simulink model "RPEM_16_12_2005prueba"  (Simulink 5.0)
settings: Solver=ode45  StartTime=0.0  StopTime=10.0  RelTol=1e-3
undefined symbols (not defined in the file): ts
libraries: simulink x5
settings Model: LastModifiedBy=LeO

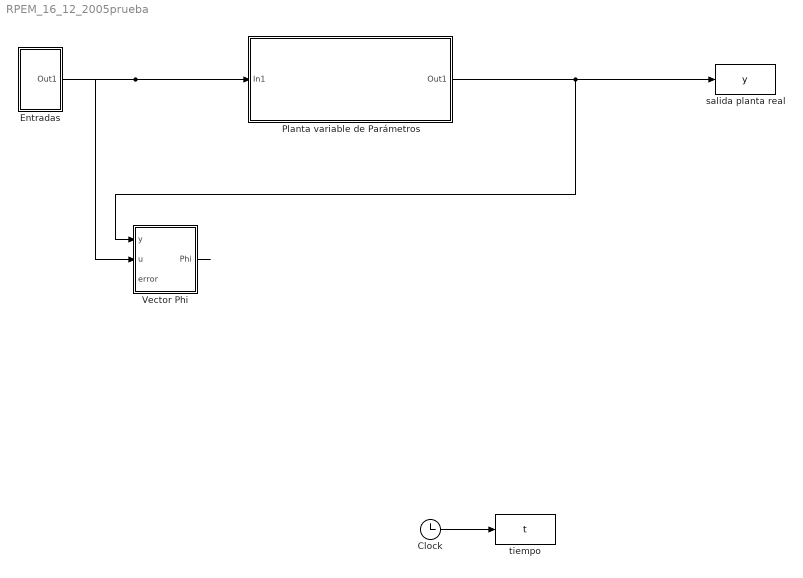
== system RPEM_16_12_2005prueba ==
  Clock : Clock
      settings: Decimation=10
  Entradas : Subsystem
  Planta variable de Parámetros : Subsystem  mask{ruido=0.05, tiempo1=40}
      mask prompts: tiempo1 "tiempo de movimiento de parametros de la planta"
  Vector Phi : Subsystem  mask{nu=1, ny=3, ne=1, nk=1}
      mask prompts: nu "Nº de u tomadas"; ny "Nº de y tomadas"; ne "Nº de errores tomados"; nk "Nº de retardo"
  salida planta real : ToWorkspace  VariableName=y  SampleTime=ts  SaveFormat=Array
  "tiempo " : ToWorkspace  VariableName=t  SampleTime=ts  SaveFormat=Array
  wires:
  Entradas/1(Out1) -> Planta variable de Parámetros/1(In1), Vector Phi/2(u)
  Clock/1 -> "tiempo "/1
  Planta variable de Parámetros/1(Out1) -> salida planta real/1, Vector Phi/1("y ")
  Vector Phi/1(Phi) -> ?

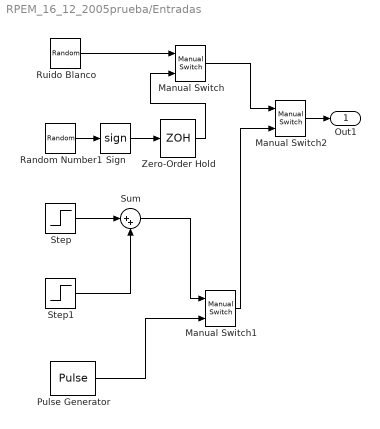
== system RPEM_16_12_2005prueba/Entradas ==
  Manual Switch : simulink/Signal Routing/Manual Switch  sw=1  action=0
  Manual Switch1 : simulink/Signal Routing/Manual Switch  sw=1  action=0
  Manual Switch2 : simulink/Signal Routing/Manual Switch  sw=1  action=0
  Pulse Generator : DiscretePulseGenerator  PulseType=Time based  PulseWidth=50
  Random Number1 : RandomNumber  SampleTime=0
  Ruido Blanco : RandomNumber  Variance=20  Seed=12  SampleTime=ts
  Sign : Signum
  Step : Step  Time=10  After=25  SampleTime=0.05
  Step1 : Step  Time=50  After=5  SampleTime=0.05
  Sum : Sum  Inputs=|++  SaturateOnIntegerOverflow=on
  Zero-Order Hold : ZeroOrderHold  SampleTime=0.05
  Out1 : Outport
  wires:
  Sign/1 -> Zero-Order Hold/1
  Random Number1/1 -> Sign/1
  Manual Switch/1 -> Manual Switch2/1
  Ruido Blanco/1 -> Manual Switch/1
  Zero-Order Hold/1 -> Manual Switch/2
  Manual Switch2/1 -> Out1/1
  Step/1 -> Sum/1
  Step1/1 -> Sum/2
  Manual Switch1/1 -> Manual Switch2/2
  Sum/1 -> Manual Switch1/1
  Pulse Generator/1 -> Manual Switch1/2

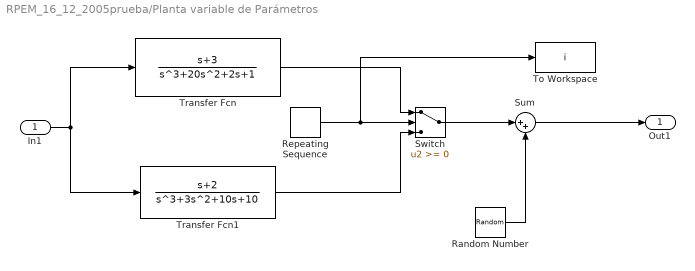
== system RPEM_16_12_2005prueba/Planta variable de Parámetros ==
  In1 : Inport
  Random Number : RandomNumber  Variance=ruido  SampleTime=0
  Repeating Sequence : simulink/Sources/Repeating Sequence  rep_seq_t=[0 2*tiempo1]  rep_seq_y=[1 -1 ]
  Sum : Sum  Inputs=|++  SaturateOnIntegerOverflow=on
  Switch : Switch  SaturateOnIntegerOverflow=on
  To Workspace : ToWorkspace  VariableName=i  SampleTime=-1  SaveFormat=Array
  Transfer Fcn : TransferFcn  Numerator=[1 3 ]  Denominator=[1 20 2 1]
  Transfer Fcn1 : TransferFcn  Numerator=[1 2]  Denominator=[1 3 10 10]
  Out1 : Outport
  wires:
  Transfer Fcn/1 -> Switch/1
  Repeating Sequence/1 -> Switch/2, To Workspace/1
  Transfer Fcn1/1 -> Switch/3
  In1/1 -> Transfer Fcn/1, Transfer Fcn1/1
  Switch/1 -> Sum/1
  Sum/1 -> Out1/1
  Random Number/1 -> Sum/2

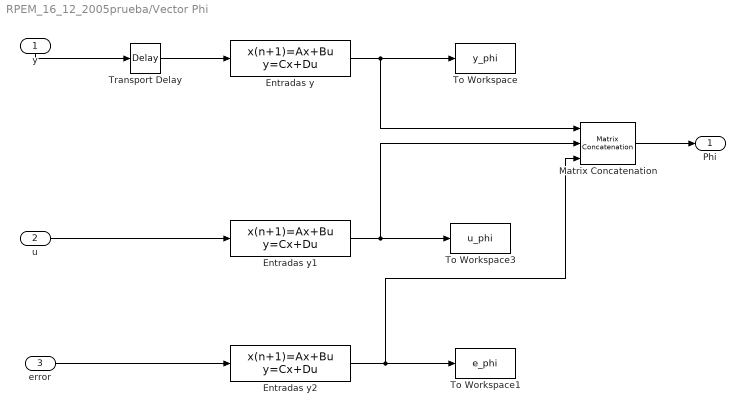
== system RPEM_16_12_2005prueba/Vector Phi ==
  "y " : Inport  Orientation=down  SampleTime=ts
  u : Inport  Port=2  SampleTime=ts
  error : Inport  Port=3  SampleTime=ts
  Entradas y : DiscreteStateSpace  A=[zeros(1,ny) ;eye(ny-1,ny)]  B=[[-1 zeros(1,ny-1)]']  C=[eye(ny)]  D=[zeros(1,ny)']  SampleTime=ts
  Entradas y1 : DiscreteStateSpace  A=[zeros(1,nu) ;eye(nu-1,nu)]  B=[[-1 zeros(1,nu-1)]']  C=[eye(nu)]  D=[zeros(1,nu)']  SampleTime=ts
  Entradas y2 : DiscreteStateSpace  A=[zeros(1,ne) ;eye(ne-1,ne)]  B=[[-1 zeros(1,ne-1)]']  C=[eye(ne)]  D=[zeros(1,ne)']  SampleTime=ts
  Matrix Concatenation : simulink/Math Operations/Matrix Concatenation  numInports=3  catMethod=Vertical
  To Workspace : ToWorkspace  VariableName=y_phi  SampleTime=ts  SaveFormat=Array
  To Workspace1 : ToWorkspace  VariableName=e_phi  SampleTime=ts  SaveFormat=Array
  To Workspace3 : ToWorkspace  VariableName=u_phi  SampleTime=ts  SaveFormat=Array
  Transport Delay : TransportDelay  DelayTime=nk*ts
  Phi : Outport
  wires:
  "y "/1 -> Transport Delay/1
  u/1 -> Entradas y1/1
  Entradas y/1 -> To Workspace/1, Matrix Concatenation/1
  Entradas y1/1 -> To Workspace3/1, Matrix Concatenation/2
  Matrix Concatenation/1 -> Phi/1
  Transport Delay/1 -> Entradas y/1
  error/1 -> Entradas y2/1
  Entradas y2/1 -> To Workspace1/1, Matrix Concatenation/3
